simulink model "tema6sim"  (R2022b)
settings: Solver=VariableStepAuto  StartTime=0.0  StopTime=30  RelTol=1e-3
values from neighbouring files (symbols this model uses):
  A = [0 1; -1/(L*c) -R/L]    [tema6.m]
  B = [0 ; 1/L]    [tema6.m]
  c = 0.001    [tema6.m]
  C = [0 , 1]    [tema6.m]
  D = 0    [tema6.m]
  L = 1    [tema6.m]
  R = 1000    [tema6.m]
libraries: simulink x1
settings Model: Creator=Fernando  LastModifiedBy=Fernando

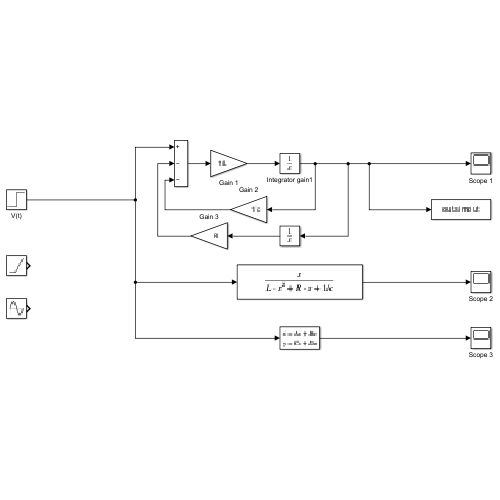
[thumbnail: Simulink's stored preview of the top-level diagram]
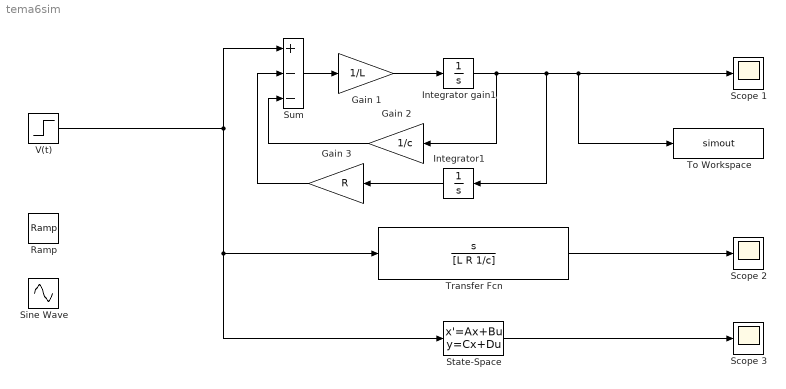
== system tema6sim ==
  Gain 1 : Gain  Gain=1/L
  Gain 2 : Gain  Gain=1/c
  Gain 3 : Gain  Gain=R
  Integrator gain1 : Integrator
  Integrator1 : Integrator
  Ramp : simulink/Sources/Ramp  slope=1  start=0  InitialOutput=0
  Scope 1 : Scope
  Scope 2 : Scope
  Scope 3 : Scope
  Sine Wave : Sin  SampleTime=0
  State-Space : StateSpace  A=A  B=B  C=C  D=D  InitialCondition=0
  Sum : Sum  Inputs=+--
  To Workspace : ToWorkspace  VariableName=simout  SaveFormat=Timeseries  SampleTime=-1
  Transfer Fcn : TransferFcn  Numerator=[1 0]  Denominator=[L R 1/c]
  V(t) : Step  SampleTime=0
  wires:
  Sum/1 -> Gain 1/1
  Gain 1/1 -> Integrator gain1/1
  Gain 2/1 -> Sum/3
  Gain 3/1 -> Sum/2
  State-Space/1 -> Scope 3/1
  Transfer Fcn/1 -> Scope 2/1
  Integrator1/1 -> Gain 3/1
  Integrator gain1/1 -> To Workspace/1, Scope 1/1, Integrator1/1, Gain 2/1
  V(t)/1 -> Sum/1, Transfer Fcn/1, State-Space/1
